simulink model "Torque"  (R2025b)
settings: Solver=VariableStepAuto  StartTime=0.0  StopTime=10.0  RelTol=1e-3
values from neighbouring files (symbols this model uses):
  B = 0.072    [parametros.m]
  emax = 1.8    [parametros.m]
  Hl = 44e6    (= 44000000)    [parametros.m]
  k1 = 1.44e5    (= 144000)    [parametros.m]
  k2 = 0.46    [parametros.m]
  k3 = 9.1e-4    (= 0.00091)    [parametros.m]
  k4 = 0.075    [parametros.m]
  kqueda = 0.001    [parametros.m]
  N = 800    [parametros.m]
  nVol = 0.85    [parametros.m]
  P_im = 40000    [parametros.m]
  pme_calculado = 1    [parametros.m]
  R = 287    [parametros.m]
  S = 0.0814    [parametros.m]
  SA = 20    [parametros.m]
  SA_MBT = 25    [parametros.m]
  sigma0 = 14.7    [parametros.m]
  V_d = 0.0013    [parametros.m]
  Vm = 300    [parametros.m]
settings Model: Creator=rebec  LastModifiedBy=rebec

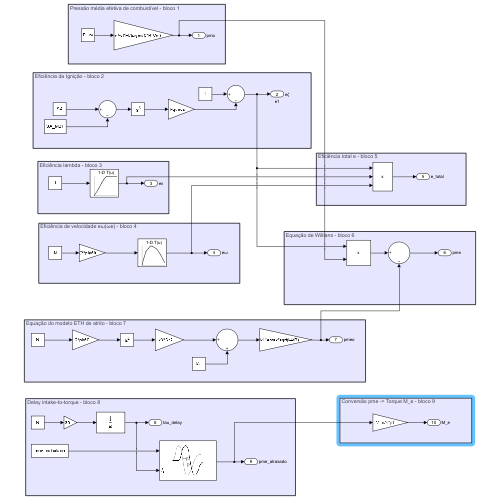
[thumbnail: Simulink's stored preview of the top-level diagram]
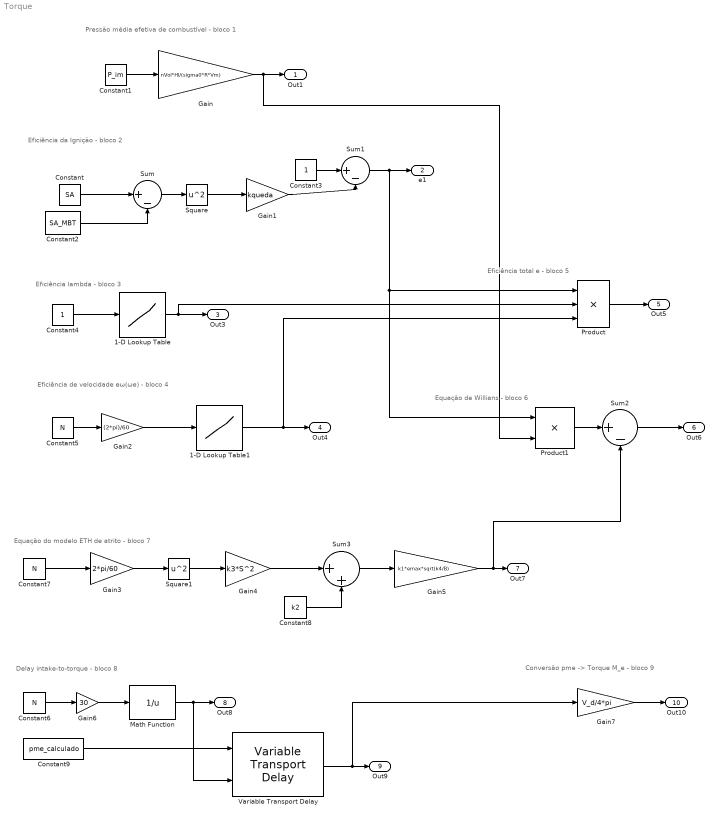
== system Torque ==
  note: Conversão pme -> Torque M_e - bloco 9
  note: Delay intake-to-torque - bloco 8
  note: Equação do modelo ETH de atrito - bloco 7
  note: Equação de Willians - bloco 6
  note: Eficiência total e - bloco 5
  note: Eficiência de velocidade eω(ωe) - bloco 4
  note: Eficiência lambda - bloco 3
  note: Eficiência da Ignição - bloco 2
  note: Pressão média efetiva de combustível - bloco 1
  1-D Lookup Table : Lookup_n-D  NumberOfTableDimensions=1  BreakpointsForDimension1=[0.70, 0.80, 0.90, 0.95, 1.00, 1.03, 1.10, 1.30]  Table=[0.59, 0.72, 0.86, 0.93, 0.98, 1.00, 1.00, 1.00]  InternalRulePriority=Speed  RndMeth=Simplest
  1-D Lookup Table1 : Lookup_n-D  NumberOfTableDimensions=1  BreakpointsForDimension1="[52,  83,  105, 157, 209, 262, 314, 419, 524, 628]"  Table=[0.28, 0.30, 0.31, 0.33, 0.34, 0.35, 0.35, 0.34, 0.32, 0.29]  InternalRulePriority=Speed  RndMeth=Simplest
  Constant : Constant  Value=SA
  Constant1 : Constant  Value=P_im
  Constant2 : Constant  Value=SA_MBT
  Constant3 : Constant
  Constant4 : Constant
  Constant5 : Constant  Value=N
  Constant6 : Constant  Value=N
  Constant7 : Constant  Value=N
  Constant8 : Constant  Value=k2
  Constant9 : Constant  Value=pme_calculado
  Gain : Gain  Gain=nVol*Hl/(sigma0*R*Vm)
  Gain1 : Gain  Gain=kqueda
  Gain2 : Gain  Gain=(2*pi)/60
  Gain3 : Gain  Gain=2*pi/60
  Gain4 : Gain  Gain=k3*S^2
  Gain5 : Gain  Gain=k1*emax*sqrt(k4/B)
  Gain6 : Gain  Gain=30
  Gain7 : Gain  Gain=V_d/4*pi
  Math Function : Math  Operator=reciprocal
  Product : Product  Inputs=3
  Product1 : Product
  Square : Math  Operator=square
  Square1 : Math  Operator=square
  Sum : Sum  Inputs=|+-
  Sum1 : Sum  Inputs=|+-
  Sum2 : Sum  Inputs=|+-
  Sum3 : Sum  Inputs=|++
  Variable Transport Delay : VariableTransportDelay  VariableDelayType=Variable transport delay  MaximumDelay=0.1
  Out1 : Outport  SignalName=pmo
  e1 : Outport  Port=2  SignalName=eζ​
  Out3 : Outport  Port=3  SignalName=eλ
  Out4 : Outport  Port=4  SignalName=eω
  Out5 : Outport  Port=5  SignalName=e_total
  Out6 : Outport  Port=6  SignalName=pme
  Out7 : Outport  Port=7  SignalName=pmeo
  Out8 : Outport  Port=8  SignalName=tau_delay
  Out9 : Outport  Port=9  SignalName=pme_atrasado
  Out10 : Outport  Port=10  SignalName=M_e
  wires:
  Constant1/1 -> Gain/1
  Constant/1 -> Sum/1
  Constant2/1 -> Sum/2
  Sum/1 -> Square/1
  Square/1 -> Gain1/1
  Constant3/1 -> Sum1/1
  Gain1/1 -> Sum1/2
  Constant4/1 -> 1-D Lookup Table/1
  1-D Lookup Table/1 -> Product/2, Out3/1
  Constant5/1 -> Gain2/1
  Gain2/1 -> 1-D Lookup Table1/1
  1-D Lookup Table1/1 -> Product/3, Out4/1
  Product/1 -> Out5/1
  Sum1/1 -> Product1/1, Product/1, e1/1
  Gain/1 -> Product1/2, Out1/1
  Product1/1 -> Sum2/1
  Sum2/1 -> Out6/1
  Constant7/1 -> Gain3/1
  Gain3/1 -> Square1/1
  Square1/1 -> Gain4/1
  Gain4/1 -> Sum3/1
  Constant8/1 -> Sum3/2
  Sum3/1 -> Gain5/1
  Gain5/1 -> Out7/1, Sum2/2
  Constant6/1 -> Gain6/1
  Gain6/1 -> Math Function/1
  Math Function/1 -> Variable Transport Delay/2, Out8/1
  Constant9/1 -> Variable Transport Delay/1
  Variable Transport Delay/1 -> Gain7/1, Out9/1
  Gain7/1 -> Out10/1
